simulink model "sim1"  (R2017a)
settings: Solver=FixedStepAuto  StartTime=0.0  StopTime=10.0  FixedStep=1/1000  RelTol=1e-3
values from neighbouring files (symbols this model uses):
  Fs = 1000    [spettrogramma.m]
undefined symbols (not defined in the file or in its folder): get, Radix
libraries: dspxfrm3 x1, dspsrcs4 x1, dspsnks4 x1
settings Model: Creator=Enrico Donato  LastModifiedBy=Enrico Donato

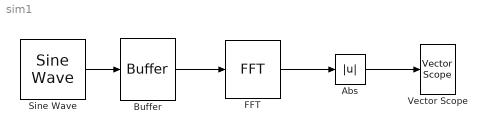
== system sim1 ==
  Abs : Abs
  Buffer : Buffer  N=1024  OutputFrames=off
  FFT : dspxfrm3/FFT  FFTImplementation=Radix-2  CompMethod=Table lookup  TableOpt=NEW  TableOptActive=Speed  BitRevOrder=off  Normalize=off  InheritFFTLength=on  FFTLength=64  WrapInput=on  roundingMode=Floor  overflowMode=off  firstCoeffDataTypeStr=Inherit: Same word length as input  firstCoeffLastDataTypeStr=Inherit: Same word length as input  outputMin=[]  outputMax=[]
  Sine Wave : dspsrcs4/Sine Wave  Amplitude=1  Frequency=100  Phase=0  SampleMode=Discrete  OutComplex=Real  CompMethod=Trigonometric fcn  TableSize=Speed  SampleTime=1/1000  SamplesPerFrame=1  ResetState=Restart at time zero  OutputFrames=off  dataType=double  wordLen=16  udDataType=sfix(16)  fracBitsMode=Best precision  numFracBits=15  OutDataTypeStr=double  LastOutDataTypeStr=double
  Vector Scope : dspsnks4/Vector Scope  ScopeProperties=on  Domain=Frequency  HorizSpan=1  DisplayProperties=off  AxisGrid=on  Memory=off  FrameNumber=on  AxisLegend=off  AxisZoom=off  OpenScopeAtSimStart=on  OpenScopeImmediately=off  FigPos=get(0,'defaultfigureposition')  AxisProperties=off  XUnits=Hertz  XRange=[-Fs/2...Fs/2]  InheritXIncr=on  XIncr=1  XLabel=Time  XLimit=Auto  XMin=0  XMax=1  XStart=0  YUnits=dB  YLabel=Amplitude  LineProperties=off  XAxisParamsVer=6.9
      settings: SourceProductName=DSP System Toolbox  SourceProductBaseCode=DS  YMin=-10  YMax=10
  wires:
  Buffer/1 -> FFT/1
  Sine Wave/1 -> Buffer/1
  FFT/1 -> Abs/1
  Abs/1 -> Vector Scope/1
